simulink model "sim_quadprog_updated_data"  (R2020b)
settings: Solver=FixedStepAuto  StartTime=0.0  StopTime=T_sim  FixedStep=dt  RelTol=1e-3
undefined symbols (not defined in the file): A_alpha1, A_init, A_TEC, b_a, b_alpha1, b_dyn, b_TEC, C, dt, H, H_a, L, lambda_alpha, lambda_beta, lb, lb_a, m, N, NOISE, noise_bound_cl, nu, p, S_y, T_Track, T_Track2, T_Track3, ub, ub_a, ud, x0, y_T1, y_T2, y_T3, y_T4, yd
libraries: simulink x5
settings Model: Creator=Fabian  LastModifiedBy=Fabian

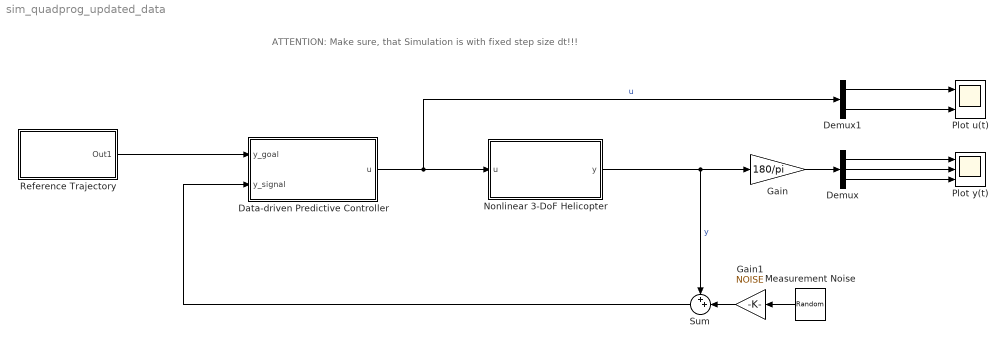
== system sim_quadprog_updated_data ==
  note: ATTENTION: Make sure, that Simulation is with fixed step size dt!!!
  Data-driven Predictive Controller : Subsystem
  Demux : Demux  Outputs=3
  Demux1 : Demux  Outputs=2
  Gain : Gain  Gain=180/pi
  Gain1 : Gain  Gain=NOISE
  Measurement Noise : UniformRandomNumber  Minimum=-noise_bound_cl  Maximum=noise_bound_cl  Seed=[3;4;5]  SampleTime=dt
  Nonlinear 3-DoF Helicopter : Subsystem
  Plot u(t) : Scope  NumInputPorts=2
  Plot y(t) : Scope  NumInputPorts=3
  Reference Trajectory : Subsystem
  Sum : Sum  Inputs=++|
  wires:
  Measurement Noise/1 -> Gain1/1
  Demux/3 -> Plot y(t)/3
  Demux/2 -> Plot y(t)/2
  Demux1/1 -> Plot u(t)/1
  Demux/1 -> Plot y(t)/1
  Demux1/2 -> Plot u(t)/2
  Gain/1 -> Demux/1
  Nonlinear 3-DoF Helicopter/1(y) -> Gain/1, Sum/1  "y"
  Data-driven Predictive Controller/1(u) -> Demux1/1, Nonlinear 3-DoF Helicopter/1(u)  "u"
  Sum/1 -> Data-driven Predictive Controller/2(y_signal)
  Reference Trajectory/1(Out1) -> Data-driven Predictive Controller/1(y_goal)
  Gain1/1 -> Sum/2

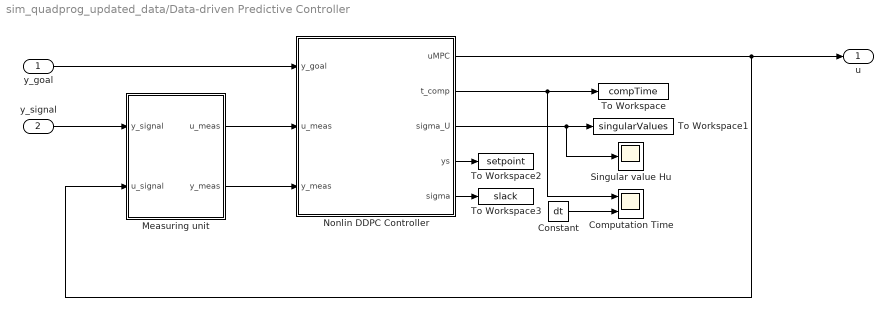
== system sim_quadprog_updated_data/Data-driven Predictive Controller ==
  y_goal : Inport
  y_signal : Inport  Port=2
  Computation Time : Scope  NumInputPorts=2
  Constant : Constant  Value=dt
  Measuring unit : Subsystem
  Nonlin DDPC Controller : MATLAB Function  TreatAsAtomicUnit=on
  Singular value Hu : Scope
  To Workspace : ToWorkspace  VariableName=compTime  SaveFormat=Timeseries  SampleTime=-1
  To Workspace1 : ToWorkspace  VariableName=singularValues  SaveFormat=Timeseries  SampleTime=-1
  To Workspace2 : ToWorkspace  VariableName=setpoint  SaveFormat=Timeseries  SampleTime=-1
  To Workspace3 : ToWorkspace  VariableName=slack  SaveFormat=Timeseries  SampleTime=-1
  u : Outport
  wires:
  y_signal/1 -> Measuring unit/1(y_signal)
  Measuring unit/1(u_meas) -> Nonlin DDPC Controller/2(u_meas)
  Measuring unit/2(y_meas) -> Nonlin DDPC Controller/3(y_meas)
  Nonlin DDPC Controller/1(uMPC) -> u/1, Measuring unit/2(u_signal)
  Nonlin DDPC Controller/2(t_comp) -> Computation Time/1, To Workspace/1
  Constant/1 -> Computation Time/2
  Nonlin DDPC Controller/3(sigma_U) -> Singular value Hu/1, To Workspace1/1
  y_goal/1 -> Nonlin DDPC Controller/1(y_goal)
  Nonlin DDPC Controller/4(ys) -> To Workspace2/1
  Nonlin DDPC Controller/5(sigma) -> To Workspace3/1

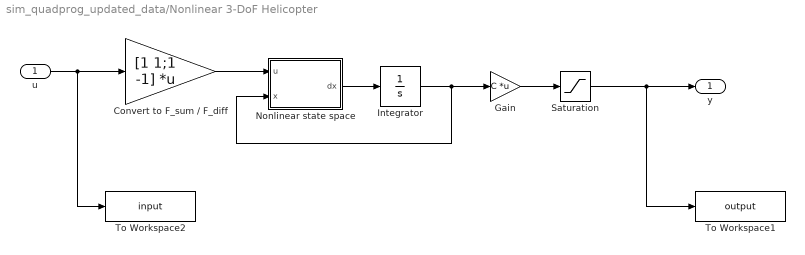
== system sim_quadprog_updated_data/Nonlinear 3-DoF Helicopter ==
  u : Inport
  Convert to F_sum / F_diff : Gain  Gain=[1 1;1 -1]  Multiplication=Matrix(K*u)
  Gain : Gain  Gain=C  Multiplication=Matrix(K*u)
  Integrator : Integrator  InitialCondition=x0
  Nonlinear state space : MATLAB Function  TreatAsAtomicUnit=on
  Saturation : Saturate  UpperLimit=[inf; 33*pi/180; 90*pi/180]  LowerLimit=[-inf; -33*pi/180; -90*pi/180]
  To Workspace1 : ToWorkspace  VariableName=output  SaveFormat=Timeseries  SampleTime=-1
  To Workspace2 : ToWorkspace  VariableName=input  SaveFormat=Timeseries  SampleTime=-1
  y : Outport
  wires:
  Nonlinear state space/1(dx) -> Integrator/1
  Integrator/1 -> Nonlinear state space/2(x), Gain/1
  u/1 -> To Workspace2/1, Convert to F_sum / F_diff/1
  Convert to F_sum / F_diff/1 -> Nonlinear state space/1(u)
  Gain/1 -> Saturation/1
  Saturation/1 -> To Workspace1/1, y/1

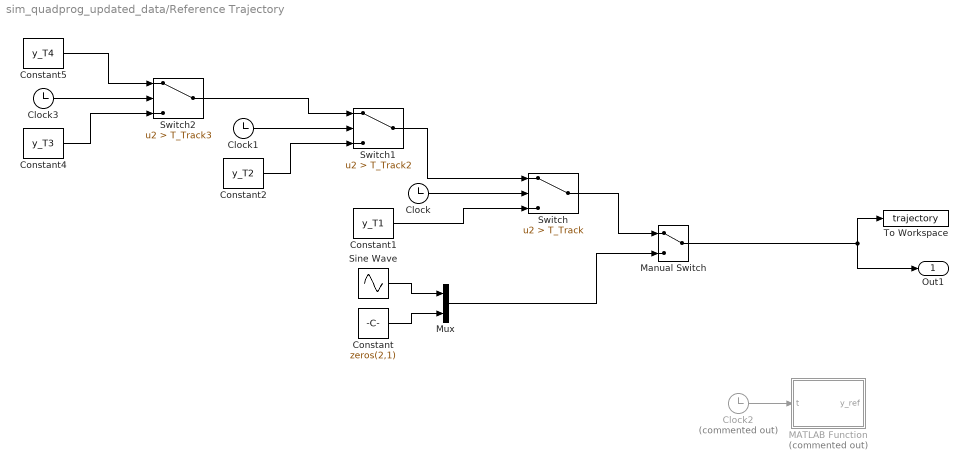
== system sim_quadprog_updated_data/Reference Trajectory ==
  Clock : Clock
  Clock1 : Clock
  Clock2 : Clock  Commented=on
  Clock3 : Clock
  Constant : Constant  Value=zeros(2,1)
  Constant1 : Constant  Value=y_T1
  Constant2 : Constant  Value=y_T2
  Constant4 : Constant  Value=y_T3
  Constant5 : Constant  Value=y_T4
  MATLAB Function : MATLAB Function  Commented=on  TreatAsAtomicUnit=on
  Manual Switch : ManualSwitch
  Mux : Mux  Inputs=2
  Sine Wave : Sin  Amplitude=45*pi/180  Frequency=2*pi*1/25  Phase=-5*2*pi*1/25  SampleTime=0
  Switch : Switch  Criteria=u2 > Threshold  Threshold=T_Track
  Switch1 : Switch  Criteria=u2 > Threshold  Threshold=T_Track2
  Switch2 : Switch  Criteria=u2 > Threshold  Threshold=T_Track3
  To Workspace : ToWorkspace  VariableName=trajectory  SaveFormat=Timeseries  SampleTime=-1
  Out1 : Outport
  wires:
  Manual Switch/1 -> Out1/1, To Workspace/1
  Switch2/1 -> Switch1/1
  Mux/1 -> Manual Switch/2
  Constant2/1 -> Switch1/3
  Clock1/1 -> Switch1/2
  Clock/1 -> Switch/2
  Sine Wave/1 -> Mux/1
  Constant/1 -> Mux/2
  Switch/1 -> Manual Switch/1
  Switch1/1 -> Switch/1
  Constant1/1 -> Switch/3
  Clock2/1 -> MATLAB Function/1(t)
  Clock3/1 -> Switch2/2
  Constant5/1 -> Switch2/1
  Constant4/1 -> Switch2/3

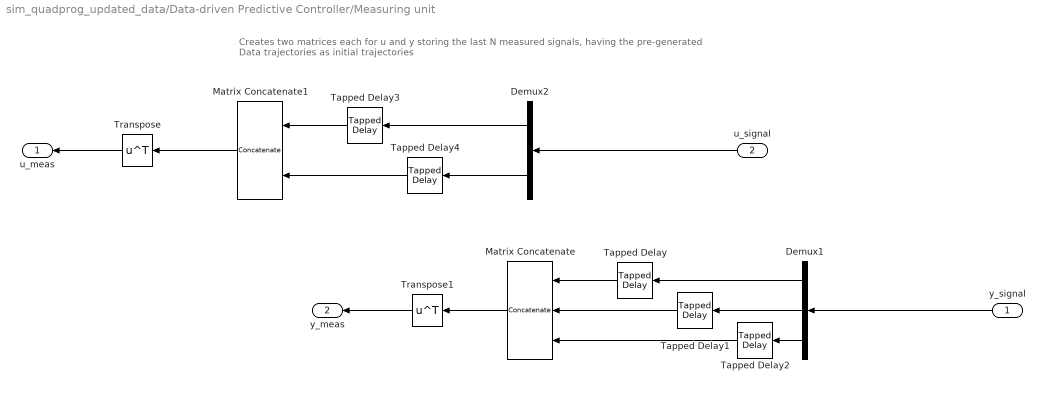
== system sim_quadprog_updated_data/Data-driven Predictive Controller/Measuring unit ==
  note: Creates two matrices each for u and y storing the last N measured signals,
      | having the pre-generated Data trajectories as initial trajectories
  y_signal : Inport
  u_signal : Inport  Port=2
  Demux1 : Demux  Outputs=3
  Demux2 : Demux  Outputs=2
  Matrix Concatenate : Concatenate  NumInputs=3  Mode=Multidimensional array  ConcatenateDimension=2
  Matrix Concatenate1 : Concatenate  Mode=Multidimensional array  ConcatenateDimension=2
  Tapped Delay : simulink/Discrete/Tapped Delay  vinit=yd(1,:)'  samptime=-1  NumDelays=N  DelayOrder=Oldest  includeCurrent=off
  Tapped Delay1 : simulink/Discrete/Tapped Delay  vinit=yd(2,:)'  samptime=-1  NumDelays=N  DelayOrder=Oldest  includeCurrent=off
  Tapped Delay2 : simulink/Discrete/Tapped Delay  vinit=yd(3,:)'  samptime=-1  NumDelays=N  DelayOrder=Oldest  includeCurrent=off
  Tapped Delay3 : simulink/Discrete/Tapped Delay  vinit=ud(1,:)'  samptime=-1  NumDelays=N  DelayOrder=Oldest  includeCurrent=off
  Tapped Delay4 : simulink/Discrete/Tapped Delay  vinit=ud(2,:)'  samptime=-1  NumDelays=N  DelayOrder=Oldest  includeCurrent=off
  Transpose : Math  Operator=transpose  SaturateOnIntegerOverflow=on
  Transpose1 : Math  Operator=transpose  SaturateOnIntegerOverflow=on
  u_meas : Outport
  y_meas : Outport  Port=2
  wires:
  Demux2/2 -> Tapped Delay4/1
  Demux2/1 -> Tapped Delay3/1
  Tapped Delay3/1 -> Matrix Concatenate1/1
  Demux1/1 -> Tapped Delay/1
  Demux1/2 -> Tapped Delay1/1
  Tapped Delay4/1 -> Matrix Concatenate1/2
  Demux1/3 -> Tapped Delay2/1
  Tapped Delay1/1 -> Matrix Concatenate/2
  Tapped Delay/1 -> Matrix Concatenate/1
  Tapped Delay2/1 -> Matrix Concatenate/3
  u_signal/1 -> Demux2/1
  y_signal/1 -> Demux1/1
  Matrix Concatenate1/1 -> Transpose/1
  Transpose/1 -> u_meas/1
  Matrix Concatenate/1 -> Transpose1/1
  Transpose1/1 -> y_meas/1

== matlab function sim_quadprog_updated_data/Reference Trajectory/MATLAB Function ==
  data: t input; y_ref output
function y_ref = fcn(t)
       

    y_home_v = [0*pi/180; 0*pi/180; 0];  
    y_cargo_v = [90*pi/180; 0*pi/180; 0]; 
    y_cargo = [90*pi/180; -22*pi/180; 0];
    y_drop_v = [450*pi/180; 0*pi/180; 0];
    y_drop = [450*pi/180; -22*pi/180; 0];
    y_home = [0*pi/180; -27*pi/180; 0];

    if (0 <= t) && t < 5
        y_ref = y_home_v;
    elseif (5 <= t) && t < 17
        y_ref = y_cargo_v;
    elseif (17 <= t) && t < 30
        y_ref = y_cargo;
    elseif (30 <= t) && t < 35
        y_ref = y_cargo_v;
    elseif (35 <= t) && t < 50
        y_ref = y_drop_v;
    elseif (50 <= t) && t < 65
        y_ref = y_drop;
    elseif (65 <= t) && t < 70
        y_ref = y_drop_v;
    elseif (70 <= t) && t < 90
        y_ref = y_home_v;
    elseif t > 90
        y_ref = y_home;
    else
        y_ref = y_home;
    end

end

== matlab function sim_quadprog_updated_data/Nonlinear 3-DoF Helicopter/Nonlinear state space ==
  data: u input; x input; dx output
function dx = fcn(u,x)

%%%%%%%%%%%%%%%%%%%%%%%%%%%%%%%%%%%%%%%%%%%%%%%%%%%%%%%%%%%%%%%%%%%%%%%%
%%%%%%%%%%%%%%%%%%%%% ATTENTION %%%%%%%%%%%%%%%%%%%%%%%%%%%%%%%%%%%%%%%%
%%%% Input is F_sum and F_diff, not F_front and F_back !! %%%%%%%%%%%%%%
%%%%%%%%%%%%%%%%%%%%%%%%%%%%%%%%%%%%%%%%%%%%%%%%%%%%%%%%%%%%%%%%%%%%%%%%

    m_H = 1.322;
    m_A = 2.638;

    Jxx = 1.1455;
    Jyy = 1.1184;
    Jzz = 0.032;

    r = 0.1775;

    rHx = -0.089;
    rHz = 0.655;
    rAHx = -0.034;
    rAHz = 0.0193;

    g = 9.81;
    
    dalph = x(2);
    bet = x(3);
    dbet = x(4);
    gam = x(5);
    dgam = x(6);
    
    Fsum = u(1);
    Fdiff = u(2);
    
    dx = [dalph;...
     1/Jxx * Fsum*sin(gam) * (rHx*sin(bet) - rHz*cos(bet));...
     dbet;...
     1/Jyy * (-(m_A+m_H)*g *(rAHz*cos(bet) - rAHx*sin(bet)) + Fsum * rHz*cos(gam));...
     dgam;...
     -1/Jzz * r * Fdiff];

end

== matlab function sim_quadprog_updated_data/Data-driven Predictive Controller/Nonlin DDPC Controller ==
  data: y_goal input; u_meas input; uMPC output; y_meas input; t_comp output; sigma_U output; H parameter; lb parameter; ub parameter; b_dyn parameter; A_init parameter; b_TEC parameter; b_alpha1 parameter; A_TEC parameter; A_alpha1 parameter; m parameter; p parameter; N parameter; L parameter; nu parameter; S_y parameter; lambda_beta parameter; ys output; H_a parameter; b_a parameter; lb_a parameter; ub_a parameter; lambda_alpha parameter; sigma output
function [uMPC, t_comp, sigma_U, ys, sigma] = fcn(y_goal, u_meas, y_meas, H, lb, ub, b_dyn, A_init, b_TEC, b_alpha1, A_TEC, A_alpha1, m, p, N, L, nu, S_y, lambda_beta, H_a, b_a, lb_a, ub_a, lambda_alpha)

    % Data-driven Model Predictive Control using Nonlinear Data with
    % instantaneous Data Update during the control process
    
    % ATTENTION: Simulation Step Size must be dt (fixed)!!!
    
    t_begin = tic; %Track computation time
    
    %% Update Hankel Matrix
    
    % Take past nu measurements for init
    u_init = u_meas(1:m, N-nu+1:N);
    y_init = y_meas(1:p, N-nu+1:N);
    
    Hu = hankel_c(u_meas(:),L,N-L+1,m);
    Hy = hankel_c(y_meas(:),L,N-L+1,p);
    
    %% Setup Quadprog
    
    %Quadprog setup
    %(Simulink coder only allows for 'Active-set' algorithm)
    coder.extrinsic('quadprog');
    options = optimoptions('quadprog','Algorithm','active-set','Display','Off');
  
    %% Set up and solve Main Quadratic Program 
    
    % Include tracking point y_goal
    f = [zeros(N-L+1,1);zeros((m+p)*L+m,1);-2*S_y*y_goal;zeros(p*L,1);-lambda_beta];
    
    % Update Dynamics with measured data
    A_dyn = [Hu -eye(m*L) zeros(m*L,p*L+m+p+p*L+1);
             Hy zeros(p*L,m*L) -eye(p*L) zeros(p*L,m+p) -eye(p*L) zeros(p*L,1)];
    
    % Update initial trajectory   
    b_init = [u_init(:); y_init(:)];
    
    A_eq = [A_dyn; A_init; A_TEC; A_alpha1];
    b_eq = [b_dyn; b_init; b_TEC; b_alpha1];

    A_ineq = [];
    b_ineq = [];
    
    %Initialize solutions
    uMPC = zeros(2,1); 
    sol_0 = zeros(N-L+1+(m+p)*L+m+p+p*L+1,1);
    
    %Solving QP
    [sol,~,~,~,~] = quadprog(H,f,A_ineq,b_ineq,A_eq,b_eq,lb,ub,sol_0,options);
    
    %Extract solution
    u_sol = sol(N-L+1+1:N-L+1+m*L);
    uMPC = u_sol(nu*m+1:nu*m+m);
    
    %%%%%%%% ATTENTION: uMPC is Front and Backmotor Force %%%%%%%%%%%%%%%%%
    
    %% Yield numeric measures
    
    t_comp = toc(t_begin);
    sigma_U = min(svd(Hu));
    
    %% Yield artificial setpoint
    
    ys = zeros(3,1);
    ys = sol((N-L+1)+(m+p)*L+m+1 : (N-L+1)+(m+p)*L+m+p);
    
    %% Yield slack
    
    sigma_vec = zeros(168,1);
    sigma_vec = sol(N-L+1+(m+p)*L+m+p+1:N-L+1+(m+p)*L+m+p+p*L);
    sigma = norm(sigma_vec);
    
end
